simulink model "RemoteMicrogrid"  (R2025a)
settings: Solver=FixedStepAuto  StartTime=0.0  StopTime=8  FixedStep=Ts  MaxStep=1e-3  RelTol=1e-3
PreLoadFcn:
  | RemoteMicrogridInputData
undefined symbols (not defined in the file): BESS, ControlRoom, DiscIntNeverNeededParam, Grid, Load, Machine, Microgrid, MicrogridStatus, PV, relay1, T_on, Ts
libraries: ee_lib x53, fl_lib x39, eeGeneralControl x30, simulink x30, nesl_utility x26, nesl_utility_internal x19, slpidlib x7, eeTransforms x5, eeRmsMeasurement x4, eeTotalHarmonicDistorsion x4, batteryecm_lib x2, simulink_extras x2
(part 3 of 6)

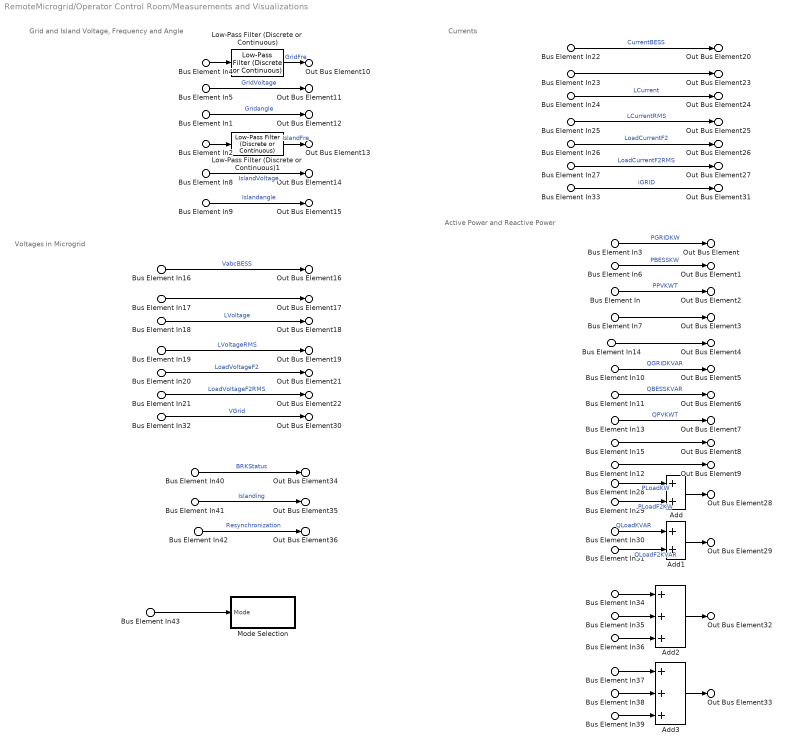
== system RemoteMicrogrid/Operator Control Room/Measurements and Visualizations  ==
  note: Currents
  note: Voltages in Microgrid
  note: Grid and Island Voltage, Frequency and Angle
  note: Active Power and Reactive Power
  Bus Element In4 : Inport  PortName=MGSubstation  Element=MGController.mPLL.Grid.frequency
  Bus Element In5 : Inport  PortName=MGSubstation  Element=MGController.mPLL.Grid.voltage
  Bus Element In1 : Inport  PortName=MGSubstation  Element=MGController.mPLL.Grid.angle
  Bus Element In2 : Inport  PortName=MGSubstation  Element=MGController.mPLL.Island.frequency
  Bus Element In8 : Inport  PortName=MGSubstation  Element=MGController.mPLL.Island.voltage
  Bus Element In9 : Inport  PortName=MGSubstation  Element=MGController.mPLL.Island.angle
  Bus Element In40 : Inport  PortName=MGSubstation  Element=MGController.BRK Status
  Bus Element In41 : Inport  PortName=MGSubstation  Element=MGController.Status.plannedIslanding
  Bus Element In42 : Inport  PortName=MGSubstation  Element=MGController.Status.resync
  Bus Element In43 : Inport  PortName=MGSubstation  Element=MGController.Status.mode
  Bus Element In10 : Inport  PortName=MGSubstation  Element=mPCC.PCC.reactivePower
  Bus Element In37 : Inport  PortName=MGSubstation  Element=mPCC.PCC.reactivePower
  Bus Element In32 : Inport  PortName=MGSubstation  Element=mPCC.PCC.voltage
  Bus Element In33 : Inport  PortName=MGSubstation  Element=mPCC.PCC.current
  Bus Element In3 : Inport  PortName=MGSubstation  Element=mPCC.PCC.activePower
  Bus Element In34 : Inport  PortName=MGSubstation  Element=mPCC.PCC.activePower
  Bus Element In6 : Inport  PortName=MGSubstation  Element=mBESS.active power
  Bus Element In35 : Inport  PortName=MGSubstation  Element=mBESS.active power
  Bus Element In11 : Inport  PortName=MGSubstation  Element=mBESS.reactive power
  Bus Element In38 : Inport  PortName=MGSubstation  Element=mBESS.reactive power
  Bus Element In16 : Inport  PortName=MGSubstation  Element=mBESS.voltage
  Bus Element In22 : Inport  PortName=MGSubstation  Element=mBESS.current
  Bus Element In : Inport  Port=2  PortName=mPV  Element=PV power.PV active power
  Bus Element In36 : Inport  Port=2  PortName=mPV  Element=PV power.PV active power
  Bus Element In13 : Inport  Port=2  PortName=mPV  Element=PV power.PV reactive power
  Bus Element In39 : Inport  Port=2  PortName=mPV  Element=PV power.PV reactive power
  Bus Element In17 : Inport  Port=2  PortName=mPV  Element=PV ac.Va
  Bus Element In23 : Inport  Port=2  PortName=mPV  Element=PV ac.Ia
  Bus Element In7 : Inport  Port=3  PortName=mLoad  Element=active power
  Bus Element In28 : Inport  Port=3  PortName=mLoad  Element=active power
  Bus Element In15 : Inport  Port=3  PortName=mLoad  Element=reactive power
  Bus Element In30 : Inport  Port=3  PortName=mLoad  Element=reactive power
  Bus Element In18 : Inport  Port=3  PortName=mLoad  Element=voltage
  Bus Element In19 : Inport  Port=3  PortName=mLoad  Element=voltageRMS
  Bus Element In24 : Inport  Port=3  PortName=mLoad  Element=current
  Bus Element In25 : Inport  Port=3  PortName=mLoad  Element=currentRMS
  Bus Element In14 : Inport  Port=4  PortName=mLoadF2  Element=active powerF2
  Bus Element In29 : Inport  Port=4  PortName=mLoadF2  Element=active powerF2
  Bus Element In12 : Inport  Port=4  PortName=mLoadF2  Element=reactive powerF2
  Bus Element In31 : Inport  Port=4  PortName=mLoadF2  Element=reactive powerF2
  Bus Element In20 : Inport  Port=4  PortName=mLoadF2  Element=voltageF2
  Bus Element In21 : Inport  Port=4  PortName=mLoadF2  Element=voltageRMSF2
  Bus Element In26 : Inport  Port=4  PortName=mLoadF2  Element=currentF2
  Bus Element In27 : Inport  Port=4  PortName=mLoadF2  Element=currentRMSF2
  Add : Sum
  Add1 : Sum
  Add2 : Sum  Inputs=+++
  Add3 : Sum  Inputs=+++
  Low-Pass Filter (Discrete or Continuous) : eeGeneralControl/Low-Pass Filter (Discrete or Continuous)  K=1  T=0.001  B=inf  A=-inf  init_option=Inherited from block input  x0=0  Ts=-1
  Low-Pass Filter (Discrete or Continuous)1 : eeGeneralControl/Low-Pass Filter (Discrete or Continuous)  K=1  T=0.001  B=inf  A=-inf  init_option=Specify as parameter  x0=0  Ts=-1
  Mode Selection : Subsystem
  Out Bus Element1 : Outport  PortName=Visualization  Element=BESS.activePower
  Out Bus Element6 : Outport  PortName=Visualization  Element=BESS.reactivePower
  Out Bus Element16 : Outport  PortName=Visualization  Element=BESS.voltage
  Out Bus Element20 : Outport  PortName=Visualization  Element=BESS.current
  Out Bus Element2 : Outport  PortName=Visualization  Element=PV.activePower
  Out Bus Element7 : Outport  PortName=Visualization  Element=PV.reactivePower
  Out Bus Element17 : Outport  PortName=Visualization  Element=PV.ACVoltage
  Out Bus Element23 : Outport  PortName=Visualization  Element=PV.ACCurrent
  Out Bus Element3 : Outport  PortName=Visualization  Element=MVLoad.activePower
  Out Bus Element8 : Outport  PortName=Visualization  Element=MVLoad.reactivePower
  Out Bus Element18 : Outport  PortName=Visualization  Element=MVLoad.voltage
  Out Bus Element19 : Outport  PortName=Visualization  Element=MVLoad.voltageRMS
  Out Bus Element24 : Outport  PortName=Visualization  Element=MVLoad.current
  Out Bus Element25 : Outport  PortName=Visualization  Element=MVLoad.currentRMS
  Out Bus Element4 : Outport  PortName=Visualization  Element=LVLoad.activePower
  Out Bus Element9 : Outport  PortName=Visualization  Element=LVLoad.reactivePower
  Out Bus Element21 : Outport  PortName=Visualization  Element=LVLoad.voltage
  Out Bus Element22 : Outport  PortName=Visualization  Element=LVLoad.voltageRMS
  Out Bus Element26 : Outport  PortName=Visualization  Element=LVLoad.current
  Out Bus Element27 : Outport  PortName=Visualization  Element=LVLoad.currentRMS
  Out Bus Element : Outport  PortName=Visualization  Element=Diesel.activePower
  Out Bus Element5 : Outport  PortName=Visualization  Element=Diesel.reactivePower
  Out Bus Element10 : Outport  PortName=Visualization  Element=Diesel.frequency
  Out Bus Element11 : Outport  PortName=Visualization  Element=Diesel.voltage
  Out Bus Element12 : Outport  PortName=Visualization  Element=Diesel.angle
  Out Bus Element13 : Outport  PortName=Visualization  Element=Island.frequency
  Out Bus Element14 : Outport  PortName=Visualization  Element=Island.voltage
  Out Bus Element15 : Outport  PortName=Visualization  Element=Island.angle
  Out Bus Element28 : Outport  PortName=Visualization  Element=Load.activePower
  Out Bus Element29 : Outport  PortName=Visualization  Element=Load.reactivePower
  Out Bus Element30 : Outport  PortName=Visualization  Element=PCC.voltage
  Out Bus Element31 : Outport  PortName=Visualization  Element=PCC.current
  Out Bus Element34 : Outport  PortName=Visualization  Element=PCC.BRKStatus
  Out Bus Element32 : Outport  PortName=Visualization  Element=Generation.activePower
  Out Bus Element33 : Outport  PortName=Visualization  Element=Generation.reactivePower
  Out Bus Element35 : Outport  PortName=Visualization  Element=plannedIslanding
  Out Bus Element36 : Outport  PortName=Visualization  Element=resynchronization
  wires:
  Bus Element In4/1 -> Low-Pass Filter (Discrete or Continuous)/1
  Bus Element In1/1 -> Out Bus Element12/1  "Gridangle"
  Bus Element In9/1 -> Out Bus Element15/1  "Islandangle"
  Bus Element In3/1 -> Out Bus Element/1  "PGRIDKW"
  Bus Element In6/1 -> Out Bus Element1/1  "PBESSKW"
  Bus Element In/1 -> Out Bus Element2/1  "PPVKWT"
  Bus Element In7/1 -> Out Bus Element3/1
  Bus Element In14/1 -> Out Bus Element4/1
  Bus Element In10/1 -> Out Bus Element5/1  "QGRIDKVAR"
  Bus Element In11/1 -> Out Bus Element6/1  "QBESSKVAR"
  Bus Element In13/1 -> Out Bus Element7/1  "QPVKWT"
  Bus Element In15/1 -> Out Bus Element8/1
  Bus Element In12/1 -> Out Bus Element9/1
  Bus Element In5/1 -> Out Bus Element11/1  "GridVoltage"
  Bus Element In2/1 -> Low-Pass Filter (Discrete or Continuous)1/1
  Bus Element In8/1 -> Out Bus Element14/1  "IslandVoltage"
  Bus Element In16/1 -> Out Bus Element16/1  "VabcBESS"
  Bus Element In17/1 -> Out Bus Element17/1
  Bus Element In18/1 -> Out Bus Element18/1  "LVoltage"
  Bus Element In19/1 -> Out Bus Element19/1  "LVoltageRMS"
  Bus Element In20/1 -> Out Bus Element21/1  "LoadVoltageF2"
  Bus Element In21/1 -> Out Bus Element22/1  "LoadVoltageF2RMS"
  Bus Element In23/1 -> Out Bus Element23/1
  Bus Element In24/1 -> Out Bus Element24/1  "LCurrent"
  Bus Element In26/1 -> Out Bus Element26/1  "LoadCurrentF2"
  Bus Element In27/1 -> Out Bus Element27/1  "LoadCurrentF2RMS"
  Bus Element In22/1 -> Out Bus Element20/1  "CurrentBESS"
  Bus Element In25/1 -> Out Bus Element25/1  "LCurrentRMS"
  Bus Element In28/1 -> Add/1  "PLoadKW"
  Bus Element In29/1 -> Add/2  "PLoadF2KW"
  Add/1 -> Out Bus Element28/1
  Add1/1 -> Out Bus Element29/1
  Bus Element In31/1 -> Add1/2  "QLoadF2KVAR"
  Bus Element In30/1 -> Add1/1  "QLoadKVAR"
  Bus Element In32/1 -> Out Bus Element30/1  "VGrid"
  Bus Element In33/1 -> Out Bus Element31/1  "iGRID"
  Bus Element In34/1 -> Add2/1
  Bus Element In35/1 -> Add2/2
  Bus Element In36/1 -> Add2/3
  Bus Element In38/1 -> Add3/2
  Bus Element In39/1 -> Add3/3
  Bus Element In37/1 -> Add3/1
  Add2/1 -> Out Bus Element32/1
  Add3/1 -> Out Bus Element33/1
  Bus Element In40/1 -> Out Bus Element34/1  "BRKStatus"
  Bus Element In41/1 -> Out Bus Element35/1  "Islanding"
  Bus Element In42/1 -> Out Bus Element36/1  "Resynchronization"
  Bus Element In43/1 -> Mode Selection/1(Mode)
  Low-Pass Filter (Discrete or Continuous)/1 -> Out Bus Element10/1  "GridFre"
  Low-Pass Filter (Discrete or Continuous)1/1 -> Out Bus Element13/1  "IslandFre"

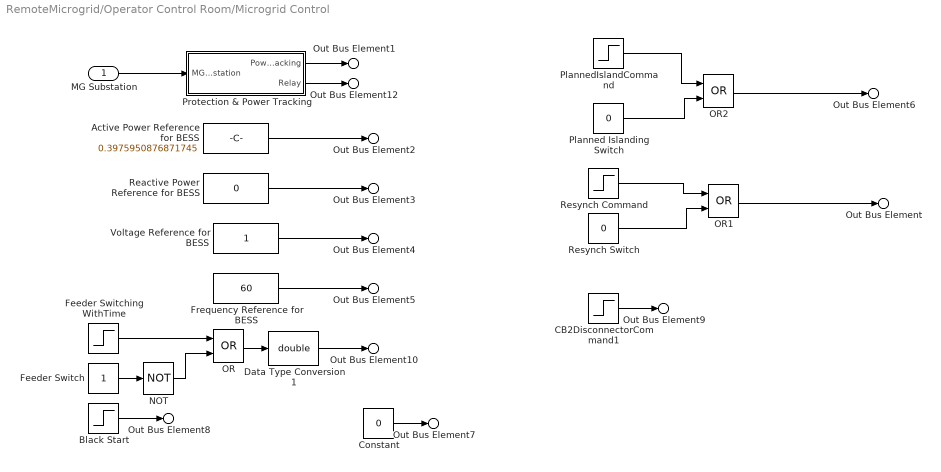
== system RemoteMicrogrid/Operator Control Room/Microgrid Control ==
  MG Substation : Inport
  Active Power Reference for BESS : Constant  Value=0.3975950876871745
  Black Start : Step  Time=100  SampleTime=Ts
  CB2DisconnectorCommand1 : Step  Time=ControlRoom.BRKControl  SampleTime=Ts
  Constant : Constant  Value=0
  Data Type Conversion1 : DataTypeConversion  OutDataTypeStr=double  SaturateOnIntegerOverflow=off  RndMeth=Floor
  Feeder Switch : Constant
  Feeder Switching WithTime : Step  Time=ControlRoom.FeederSwitchTime  SampleTime=Ts
  Frequency Reference for BESS : Constant  Value=60
  NOT : Logic  Operator=NOT  IconShape=distinctive  AllPortsSameDT=off  OutDataTypeStr=boolean
  OR : Logic  Operator=OR  AllPortsSameDT=off  OutDataTypeStr=boolean
  OR1 : Logic  Operator=OR  AllPortsSameDT=off  OutDataTypeStr=boolean
  OR2 : Logic  Operator=OR  AllPortsSameDT=off  OutDataTypeStr=boolean
  Planned Islanding Switch : Constant  Value=0
  PlannedIslandCommand : Step  Time=ControlRoom.PlannedIsland  SampleTime=Ts
  Protection & Power Tracking : Subsystem
  Reactive Power Reference for BESS : Constant  Value=0
  Resynch Command : Step  Time=ControlRoom.Resynch  SampleTime=Ts
  Resynch Switch : Constant  Value=0
  Voltage Reference for BESS : Constant
  Out Bus Element6 : Outport  PortName=CtrlRmSubstation  Element=PlannedIslandCmd
  Out Bus Element9 : Outport  PortName=CtrlRmSubstation  Element=BRKcontrol
  Out Bus Element : Outport  PortName=CtrlRmSubstation  Element=ResynchCmd
  Out Bus Element1 : Outport  PortName=CtrlRmSubstation  Element=PowerCmd
  Out Bus Element2 : Outport  PortName=CtrlRmSubstation  Element=Pref
  Out Bus Element3 : Outport  PortName=CtrlRmSubstation  Element=Qref
  Out Bus Element8 : Outport  PortName=CtrlRmSubstation  Element=BlackStart
  Out Bus Element4 : Outport  PortName=CtrlRmSubstation  Element=Vref
  Out Bus Element5 : Outport  PortName=CtrlRmSubstation  Element=Fref
  Out Bus Element7 : Outport  PortName=CtrlRmSubstation  Element=BESSReactivePower
  Out Bus Element12 : Outport  PortName=CtrlRmSubstation  Element=UnplannedIslanding
  Out Bus Element10 : Outport  Port=2  PortName=CtrlRmFeeder  Element=FeederSwitch
  wires:
  Data Type Conversion1/1 -> Out Bus Element10/1
  Resynch Command/1 -> OR1/1
  OR/1 -> Data Type Conversion1/1
  Active Power Reference for BESS/1 -> Out Bus Element2/1
  PlannedIslandCommand/1 -> OR2/1
  Planned Islanding Switch/1 -> OR2/2
  Resynch Switch/1 -> OR1/2
  Feeder Switching WithTime/1 -> OR/1
  Protection & Power Tracking/1(Power tracking) -> Out Bus Element1/1
  Feeder Switch/1 -> NOT/1
  CB2DisconnectorCommand1/1 -> Out Bus Element9/1
  MG Substation/1 -> Protection & Power Tracking/1(MGSubstation)
  OR2/1 -> Out Bus Element6/1
  Black Start/1 -> Out Bus Element8/1
  Voltage Reference for BESS/1 -> Out Bus Element4/1
  Frequency Reference for BESS/1 -> Out Bus Element5/1
  Constant/1 -> Out Bus Element7/1
  NOT/1 -> OR/2
  OR1/1 -> Out Bus Element/1
  Protection & Power Tracking/2(Relay) -> Out Bus Element12/1
  Reactive Power Reference for BESS/1 -> Out Bus Element3/1

== system RemoteMicrogrid/Operator Control Room/Performance and Power Quality ==
  Bus Element In4 : Inport  PortName=Visualization  Element=MVLoad.voltage
  Bus Element In5 : Inport  PortName=Visualization  Element=MVLoad.current
  Bus Element In7 : Inport  PortName=Visualization  Element=MVLoad.voltageRMS
  Bus Element In8 : Inport  PortName=Visualization  Element=MVLoad.currentRMS
  Bus Element In9 : Inport  PortName=Visualization  Element=MVLoad.activePower
  Bus Element In1 : Inport  PortName=Visualization  Element=PCC.voltage
  Bus Element In6 : Inport  PortName=Visualization  Element=PCC.current
  Bus Element In2 : Inport  PortName=Visualization  Element=Island.frequency
  Bus Element In3 : Inport  PortName=Visualization  Element=Island.voltage
  Bus Element In10 : Inport  PortName=Visualization  Element=Generation.activePower
  Bus Element In11 : Inport  PortName=Visualization  Element=Generation.reactivePower
  Bus Element In12 : Inport  PortName=Visualization  Element=Load.activePower
  Bus Element In13 : Inport  PortName=Visualization  Element=Load.reactivePower
  "Load Performance " : Subsystem
  Loss Calculation : Subsystem
  "Microgrid Power Quality " : Subsystem
  THD : Subsystem
  wires:
  Bus Element In4/1 -> THD/1(LoadVoltage)
  Bus Element In5/1 -> THD/2(LoadCurrent)
  Bus Element In1/1 -> THD/3(PCCVoltage)
  Bus Element In6/1 -> THD/4(PCCCurrent)
  Bus Element In2/1 -> "Microgrid Power Quality "/1(Frequency)
  Bus Element In3/1 -> "Microgrid Power Quality "/2(Voltage)
  Bus Element In7/1 -> "Load Performance "/1(VRMS)
  Bus Element In8/1 -> "Load Performance "/2(IRMS)
  Bus Element In9/1 -> "Load Performance "/3(Active Power)
  Bus Element In10/1 -> Loss Calculation/1(Active Power Gen)
  Bus Element In11/1 -> Loss Calculation/2(Reactive Power Gen)
  Bus Element In12/1 -> Loss Calculation/3(Active Power Load)
  Bus Element In13/1 -> Loss Calculation/4(Reactive Power Load)

== system RemoteMicrogrid/PV /30 kW PV ==
  In Bus Element : Inport  PortName=PV
  Current and Voltage Sensor (Three-Phase)2 : ee_lib/Sensors & Transducers/Current and Voltage Sensor (Three-Phase)  vMeasurementType=ee.enum.vmeasurement.lg  outputUnit=ee.enum.unit.pu  SRated=PV.MVA_base_new A*V  VRated=PV.KV_base_new V  I_specify=off  I_priority=None  I=[0, 0, 0] A  I_nominal_specify=off  I_nominal_value=1  I_nominal_unit=A  V_specify=off  V_priority=None  V=[0, 0, 0] V  V_nominal_specify=off  V_nominal_value=1  V_nominal_unit=V
      settings: InternalSimscapePortConfiguration="{\"Bottom\":[],\"Left\":[{\"id\":\"N1\",\"label\":\"~1\",\"type\":\"foundation.electrical.three_phase\"}],\"Right\":[{\"id\":\"V_output\",\"label\":\"V\",\"type\":\"output\"},{\"id\":\"I_output\",\"label\":\"I\",\"type\":\"output\"},{\"id\":\"N2\",\"label\":\"~2\",\"type\":\"foundation.electrical.three_phase\"}],\"Top\":[]}"
  L Filter1 : Subsystem
  Measurement1 : Subsystem
  PS-Simulink Converter1 : nesl_utility/PS-Simulink Converter  PhysicalDomain=network_engine_domain  SubClassName=ps_output  LeftPortType=input  RightPortType=output  PseudoPeriodic=off  Frequencies=[]  VectorFormat=inherit  Unit=inherit  AffineConversion=off
  PS-Simulink Converter3 : nesl_utility/PS-Simulink Converter  PhysicalDomain=network_engine_domain  SubClassName=ps_output  LeftPortType=input  RightPortType=output  PseudoPeriodic=off  Frequencies=[]  VectorFormat=inherit  Unit=inherit  AffineConversion=off
  PV Inverter 2 : Subsystem
  Terminator : Terminator
  ~ : PMIOPort  Side=Left
  PV power : Outport
  wires:
  PS-Simulink Converter3/1 -> Terminator/1
  In Bus Element/1 -> PV Inverter 2/1(PV)
  Measurement1/1(ipv1) -> PV Inverter 2/2(ipv1)
  PV Inverter 2/1(PV power) -> PV power/1
  PS-Simulink Converter1/1 -> Measurement1/1(u)
  connections:
  PV Inverter 2/RConn1 -- L Filter1/LConn1
  PS-Simulink Converter3/LConn1 -- Current and Voltage Sensor (Three-Phase)2/RConn1
  PS-Simulink Converter1/LConn1 -- Current and Voltage Sensor (Three-Phase)2/RConn2
  ~/RConn1 -- Current and Voltage Sensor (Three-Phase)2/RConn3
  Current and Voltage Sensor (Three-Phase)2/LConn1 -- L Filter1/RConn1

== system RemoteMicrogrid/PV /PLL & Measurements ==
  V : Inport
  Measurement2 : Subsystem
  Subsystem : Subsystem
  Out Bus Element : Outport  PortName=PV  Element=Vq
  Out Bus Element1 : Outport  PortName=PV  Element=Vd
  Out Bus Element2 : Outport  PortName=PV  Element=w
  Out Bus Element3 : Outport  PortName=PV  Element=Theta
  Out Bus Element4 : Outport  PortName=PV  Element=Vmag
  wires:
  V/1 -> Measurement2/1(u)
  Subsystem/2(freq) -> Out Bus Element2/1
  Subsystem/5(Vq) -> Out Bus Element/1
  Subsystem/3(angle) -> Out Bus Element3/1
  Subsystem/4(Vd) -> Out Bus Element1/1
  Measurement2/1(Vg) -> Subsystem/1(abc)
  Subsystem/1(mag) -> Out Bus Element4/1

== system RemoteMicrogrid/Diesel Substation, BESS, & Microgrid Controller/BESS and Controller/BESS ==
  Average-Value Voltage Source Converter (Three-Phase) : ee_lib/Semiconductors & Converters/Converters/Average-Value Voltage Source Converter (Three-Phase)  port_option=ee.enum.threePhasePort.expanded  frequency_option=ee.enum.converters.frequency.variable  input_option=ee.enum.converters.inputOption.ModWave  FRated=60 Hz  losses_parameterization=ee.enum.converters.losses.fixed  Pfixed=1 W  ks=0.01  kc1=1.7 V  kc2=0.01 Ohm  Ploss_vect=[100, 800, 1870, 3250, 4900] W  Irms_vect=[10, 100, 200, 300, 400] A  Vdc_nom=300 V  thermal_mass=30000 J/K  temperature_specify=off  temperature_priority=High  temperature=298.15 K  temperature_nominal_specify=off  temperature_nominal_value=1  temperature_nominal_unit=K
      settings: InternalSimscapePortConfiguration="{\"Bottom\":[],\"Left\":[{\"id\":\"ModWave\",\"label\":\"ModWave\",\"type\":\"input\"},{\"id\":\"a\",\"label\":\"a\",\"type\":\"foundation.electrical.electrical\"},{\"id\":\"b\",\"label\":\"b\",\"type\":\"foundation.electrical.electrical\"},{\"id\":\"c\",\"label\":\"c\",\"type\":\"foundation.electrical.electrical\"}],\"Right\":[{\"id\":\"p\",\"label\":\"+\",\"type\":\"foundation.electrical.electrical\"},{\"id\":\"n\",\"label\":\"-\",\"type\":\"foundation.electrical.electrical\"}],\"Top\":[]}"
  Battery : batteryecm_lib/Battery  Vnom=BESS.Vdc V  prm_dir=simscape.enum.battery.prm_dir.disabled  R1_dis=2 Ohm  R1_ch=2 Ohm  R1=BESS.Rs Ohm  prm_AH=simscape.enum.battery.prm_AH.infinite  AH=50 A*hr  V1=11.5 V  AH1=25 A*hr  prm_R2=simscape.enum.battery.prm_R2.disabled  R2=2000 Ohm  Tmeas=298.15 K  charge_measurement_port=simscape.enum.battery.enable.no  prm_dyn=simscape.enum.battery.prm_dyn.off  Rp1=0.005 Ohm  tau1=30 s  Rp2=0.005 Ohm  tau2=30 s  Rp3=0.005 Ohm  tau3=30 s  Rp4=0.005 Ohm  tau4=30 s  Rp5=0.005 Ohm  tau5=30 s  prm_fade=simscape.enum.battery.prm_fade.disabled  N_fade=100  AH_fade=45 A*hr  R1_fade=2.02 Ohm  R1_ch_fade=2.02 Ohm  V1_fade=10.35 V  prm_age=simscape.enum.battery.prm_age.disabled  prm_age_OCV=simscape.enum.battery.prm_age_OCV.OCV  OCV_age=0.9  SOC_age=60  Tmeas_age=298.15 K  delta_time_age_vec=[0] d  temperature_age_vec=[273] K  OCV_scaling_age=2.2134e6  OCV_offset_age=1.632e6  temp_exp_age=0.515833569 V  t_exp_age=0.75  Vnom_T2=12 V  R1_T2=2.2 Ohm  R1_T2_dis=2.2 Ohm  R1_T2_ch=2.2 Ohm  V1_T2=11.4 V  R2_T2=2200 Ohm  Rp1_T2=0.005 Ohm  tau1_T2=30 s  Rp2_T2=0.005 Ohm  tau2_T2=30 s  Rp3_T2=0.005 Ohm  tau3_T2=30 s  Rp4_T2=0.005 Ohm  tau4_T2=30 s  Rp5_T2=0.005 Ohm  tau5_T2=30 s  Tmeas2=273.15 K  thermal_port=simscape.enum.thermaleffects.omit  thermal_mass=30000 J/K  i_specify=off  i_priority=None  i=0 A  i_nominal_specify=off  i_nominal_value=1  i_nominal_unit=A  v_specify=off  v_priority=None  v=0 V  v_nominal_specify=off  v_nominal_value=1  v_nominal_unit=V  charge_specify=off  charge_priority=High  charge=50 A*hr  charge_nominal_specify=off  charge_nominal_value=1  charge_nominal_unit=A*hr  num_cycles_specify=off  num_cycles_priority=High  num_cycles=0  num_cycles_nominal_specify=off  num_cycles_nominal_value=1  num_cycles_nominal_unit=1  temperature_specify=off  temperature_priority=High  temperature=298.15 K  temperature_nominal_specify=off  temperature_nominal_value=1  temperature_nominal_unit=K
  Battery1 : batteryecm_lib/Battery  Vnom=BESS.Vdc V  prm_dir=simscape.enum.battery.prm_dir.disabled  R1_dis=2 Ohm  R1_ch=2 Ohm  R1=BESS.Rs Ohm  prm_AH=simscape.enum.battery.prm_AH.infinite  AH=50 A*hr  V1=11.5 V  AH1=25 A*hr  prm_R2=simscape.enum.battery.prm_R2.disabled  R2=2000 Ohm  Tmeas=298.15 K  charge_measurement_port=simscape.enum.battery.enable.no  prm_dyn=simscape.enum.battery.prm_dyn.off  Rp1=0.005 Ohm  tau1=30 s  Rp2=0.005 Ohm  tau2=30 s  Rp3=0.005 Ohm  tau3=30 s  Rp4=0.005 Ohm  tau4=30 s  Rp5=0.005 Ohm  tau5=30 s  prm_fade=simscape.enum.battery.prm_fade.disabled  N_fade=100  AH_fade=45 A*hr  R1_fade=2.02 Ohm  R1_ch_fade=2.02 Ohm  V1_fade=10.35 V  prm_age=simscape.enum.battery.prm_age.disabled  prm_age_OCV=simscape.enum.battery.prm_age_OCV.OCV  OCV_age=0.9  SOC_age=60  Tmeas_age=298.15 K  delta_time_age_vec=[0] d  temperature_age_vec=[273] K  OCV_scaling_age=2.2134e6  OCV_offset_age=1.632e6  temp_exp_age=0.515833569 V  t_exp_age=0.75  Vnom_T2=12 V  R1_T2=2.2 Ohm  R1_T2_dis=2.2 Ohm  R1_T2_ch=2.2 Ohm  V1_T2=11.4 V  R2_T2=2200 Ohm  Rp1_T2=0.005 Ohm  tau1_T2=30 s  Rp2_T2=0.005 Ohm  tau2_T2=30 s  Rp3_T2=0.005 Ohm  tau3_T2=30 s  Rp4_T2=0.005 Ohm  tau4_T2=30 s  Rp5_T2=0.005 Ohm  tau5_T2=30 s  Tmeas2=273.15 K  thermal_port=simscape.enum.thermaleffects.omit  thermal_mass=30000 J/K  i_specify=off  i_priority=None  i=0 A  i_nominal_specify=off  i_nominal_value=1  i_nominal_unit=A  v_specify=off  v_priority=None  v=0 V  v_nominal_specify=off  v_nominal_value=1  v_nominal_unit=V  charge_specify=off  charge_priority=High  charge=50 A*hr  charge_nominal_specify=off  charge_nominal_value=1  charge_nominal_unit=A*hr  num_cycles_specify=off  num_cycles_priority=High  num_cycles=0  num_cycles_nominal_specify=off  num_cycles_nominal_value=1  num_cycles_nominal_unit=1  temperature_specify=off  temperature_priority=High  temperature=298.15 K  temperature_nominal_specify=off  temperature_nominal_value=1  temperature_nominal_unit=K
  DC Voltage Source : fl_lib/Electrical/Electrical Sources/DC Voltage Source  Commented=on  v0=BESS.Vdc*2 V
  Electrical Reference : fl_lib/Electrical/Electrical Elements/Electrical Reference  Commented=on
  Electrical Reference4 : fl_lib/Electrical/Electrical Elements/Electrical Reference
  Phase Splitter : ee_lib/Connectors & References/Phase Splitter
  Voltage Sensor : fl_lib/Electrical/Electrical Sensors/Voltage Sensor  Commented=on
  Modulation : PMIOPort  Side=Left
  ~ : PMIOPort  Port=2  Side=Left
  connections:
  Battery/LConn1 -- Voltage Sensor/LConn1 -- DC Voltage Source/LConn1 -- Average-Value Voltage Source Converter (Three-Phase)/RConn1
  Battery/RConn1 -- Electrical Reference4/LConn1 -- Battery1/LConn1
  Phase Splitter/RConn3 -- Average-Value Voltage Source Converter (Three-Phase)/LConn4
  Battery1/RConn1 -- Voltage Sensor/RConn2 -- Electrical Reference/LConn1 -- DC Voltage Source/RConn1 -- Average-Value Voltage Source Converter (Three-Phase)/RConn2
  Phase Splitter/RConn1 -- Average-Value Voltage Source Converter (Three-Phase)/LConn2
  Modulation/RConn1 -- Average-Value Voltage Source Converter (Three-Phase)/LConn1
  Phase Splitter/RConn2 -- Average-Value Voltage Source Converter (Three-Phase)/LConn3
  Phase Splitter/LConn1 -- ~/RConn1

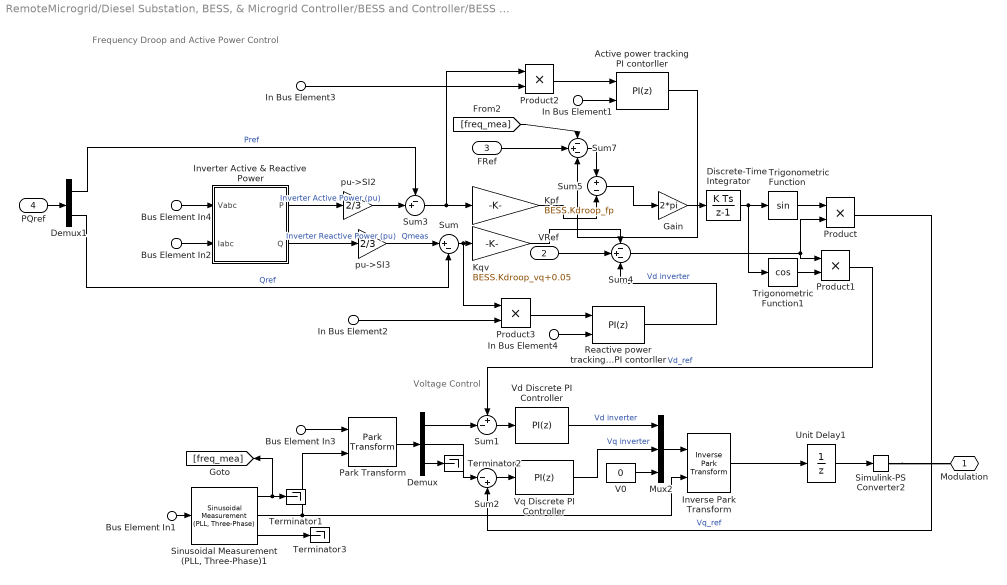
== system RemoteMicrogrid/Diesel Substation, BESS, & Microgrid Controller/BESS and Controller/BESS Control ==
  note: Frequency Droop and Active Power Control
  note: Voltage Control
  Bus Element In1 : Inport  PortName=mBESS  Element=voltage
  Bus Element In3 : Inport  PortName=mBESS  Element=voltage
  Bus Element In4 : Inport  PortName=mBESS  Element=voltage
  Bus Element In2 : Inport  PortName=mBESS  Element=current
  VRef : Inport  Port=2
  FRef : Inport  Port=3
  PQref : Inport  Port=4
  In Bus Element2 : Inport  Port=5  PortName=CntrlRmSubstation  Element=PowerCmd
  In Bus Element3 : Inport  Port=5  PortName=CntrlRmSubstation  Element=PowerCmd
  In Bus Element1 : Inport  Port=5  PortName=CntrlRmSubstation  Element=UnplannedIslanding
  In Bus Element4 : Inport  Port=5  PortName=CntrlRmSubstation  Element=UnplannedIslanding
  Active power tracking PI contorller : slpidlib/PID Controller  Controller=PI  Form=Parallel  TimeDomain=Discrete-time  UseExternalTs=off  SampleTime=Ts  IntegratorMethod=Forward Euler  FilterMethod=Forward Euler  ControllerParametersSource=internal  P=Kp_P  I=Ki_P  UseKiTs=off  D=0  UseExternalDerivativeSource=off  N=100  UseFilter=on  TunerSelectOption=Transfer Function Based (PID Tuner App)  ZeroCross=off  InitialConditionSource=internal  InitialConditionForIntegrator=BESS.Kp_0*0  InitialConditionForFilter=0  DifferentiatorICPrevScaledInput=0  ExternalReset=rising  TrackingMode=off  Kt=1  LimitOutput=off  SatLimitsSource=internal  UpperSaturationLimit=0.2  LowerSaturationLimit=-0.2  LinearizeAsGain=on  AntiWindupMode=none  Kb=1  LimitIntegrator=off  UpperIntegratorSaturationLimit=inf  LowerIntegratorSaturationLimit=-inf  POutMin=[]  POutMax=[]  IOutMin=[]  IOutMax=[]  DOutMin=[]  DOutMax=[]  NOutMin=[]  NOutMax=[]  SumOutMin=[]  SumOutMax=[]  SaturationOutMin=[]  SaturationOutMax=[]  PParamMin=[]  PParamMax=[]  IParamMin=[]  IParamMax=[]  DParamMin=[]  DParamMax=[]  NParamMin=[]  NParamMax=[]  KbParamMin=[]  KbParamMax=[]  KtParamMin=[]  KtParamMax=[]  KbOutMin=[]  KbOutMax=[]  KtOutMin=[]  KtOutMax=[]  IntegratorOutMin=[]  IntegratorOutMax=[]  FilterOutMin=[]  FilterOutMax=[]  SumI1OutMin=[]  SumI1OutMax=[]  SumI2OutMin=[]  SumI2OutMax=[]  SumI3OutMin=[]  SumI3OutMax=[]  SumI4OutMin=[]  SumI4OutMax=[]  SumDOutMin=[]  SumDOutMax=[]  DifferentiatorOutMin=[]  DifferentiatorOutMax=[]  FilterDiffOutCoefMin=[]  FilterDiffOutCoefMax=[]  ReciprocalOutMin=[]  ReciprocalOutMax=[]  SumDenOutMin=[]  SumDenOutMax=[]  SumNumOutMin=[]  SumNumOutMax=[]  DivideOutMin=[]  DivideOutMax=[]  UdiffTsProdOutMin=[]  UdiffTsProdOutMax=[]  NTsProdOutMin=[]  NTsProdOutMax=[]  UintegralTsProdOutMin=[]  UintegralTsProdOutMax=[]  UngainTsProdOutMin=[]  UngainTsProdOutMax=[]  ClampingZeroOutDataTypeStr=Inherit: Inherit via back propagation  ClampingZeroOutMin=[]  ClampingZeroOutMax=[]  FilterDenConstantOutDataTypeStr=Inherit: Inherit via back propagation  FilterDenConstantOutMin=[]  FilterDenConstantOutMax=[]  PCopyOutDataTypeStr=Inherit: Inherit via back propagation  PCopyOutMin=[]  PCopyOutMax=[]  NCopyOutDataTypeStr=Inherit: Inherit via back propagation  NCopyOutMin=[]  NCopyOutMax=[]  IntegratorContinuousStateAttributes=''  IntegratorStateMustResolveToSignalObject=off  IntegratorRTWStateStorageClass=Auto  FilterContinuousStateAttributes=''  FilterStateMustResolveToSignalObject=off  FilterRTWStateStorageClass=Auto  ParallelPVariant=InternalParameters  IdealPVariant=Disabled  IVariant=InternalParameters  DVariant=Disabled  IntegratorVariant=Discrete  SatVariant=Disabled  AWVariant=Passthrough  PCopyVariant=Disabled  TRVariant=Disabled  FdbkBlocksVariant=Forward  IdealPFdbkVariant=Disabled  SatFdbkVariant=Disabled  DerivativeFilterVariant=Disabled  NVariant=Disabled  NCopyVariant=Disabled_SignalSpec  FilterICVariant=Disabled  IntegratorICVariant=InternalICs  ExternalResetVariant=ExternalReset  TRSumVariant=Passthrough  SumFdbkVariant=Disabled  SumVariant=Sum_PI  TsampFilterVariant=InternalTs  TsampNgainVariant=Passthrough  TsampIntegralVariant=Disabled_SignalSpec  ExternalSaturationOutDataTypeStr=Inherit: Same as second input  DerivativeSourceVariant=Disabled  PreIntVariant=InternalPreInt
  Demux : Demux  Outputs=3
  Demux1 : Demux  Outputs=2
  Discrete-Time Integrator : DiscreteIntegrator  SampleTime=Ts  ICPrevOutput=DiscIntNeverNeededParam  ICPrevScaledInput=DiscIntNeverNeededParam
  Gain : Gain  Gain=2*pi
  Inverse Park Transform : eeTransforms/Inverse Park Transform  AxisAlignment=Q-axis  PowerInvariant=off
  "Inverter Active & Reactive Power " : Subsystem
  Kpf : Gain  Gain=BESS.Kdroop_fp
  Kqv : Gain  Gain=BESS.Kdroop_vq+0.05
  Mux2 : Mux  Inputs=3
  Park Transform : eeTransforms/Park Transform  AxisAlignment=Q-axis  PowerInvariant=off
  Product{,1..3} (4 alike) : Product
  Reactive power tracking PI contorller : slpidlib/PID Controller  Controller=PI  Form=Parallel  TimeDomain=Discrete-time  UseExternalTs=off  SampleTime=Ts  IntegratorMethod=Forward Euler  FilterMethod=Forward Euler  ControllerParametersSource=internal  P=Kp_Q  I=Ki_Q  UseKiTs=off  D=0  UseExternalDerivativeSource=off  N=100  UseFilter=on  TunerSelectOption=Transfer Function Based (PID Tuner App)  InitialConditionSource=internal  InitialConditionForIntegrator=BESS.Kq_0  InitialConditionForFilter=0  DifferentiatorICPrevScaledInput=0  ExternalReset=rising  TrackingMode=off  Kt=1  LimitOutput=off  SatLimitsSource=internal  UpperSaturationLimit=1.2  LowerSaturationLimit=0  LinearizeAsGain=on  AntiWindupMode=none  Kb=1  LimitIntegrator=off  UpperIntegratorSaturationLimit=inf  LowerIntegratorSaturationLimit=-inf  POutMin=[]  POutMax=[]  IOutMin=[]  IOutMax=[]  DOutMin=[]  DOutMax=[]  NOutMin=[]  NOutMax=[]  SumOutMin=[]  SumOutMax=[]  SaturationOutMin=[]  SaturationOutMax=[]  PParamMin=[]  PParamMax=[]  IParamMin=[]  IParamMax=[]  DParamMin=[]  DParamMax=[]  NParamMin=[]  NParamMax=[]  KbParamMin=[]  KbParamMax=[]  KtParamMin=[]  KtParamMax=[]  KbOutMin=[]  KbOutMax=[]  KtOutMin=[]  KtOutMax=[]  IntegratorOutMin=[]  IntegratorOutMax=[]  FilterOutMin=[]  FilterOutMax=[]  SumI1OutMin=[]  SumI1OutMax=[]  SumI2OutMin=[]  SumI2OutMax=[]  SumI3OutMin=[]  SumI3OutMax=[]  SumI4OutMin=[]  SumI4OutMax=[]  SumDOutMin=[]  SumDOutMax=[]  DifferentiatorOutMin=[]  DifferentiatorOutMax=[]  FilterDiffOutCoefMin=[]  FilterDiffOutCoefMax=[]  ReciprocalOutMin=[]  ReciprocalOutMax=[]  SumDenOutMin=[]  SumDenOutMax=[]  SumNumOutMin=[]  SumNumOutMax=[]  DivideOutMin=[]  DivideOutMax=[]  UdiffTsProdOutMin=[]  UdiffTsProdOutMax=[]  NTsProdOutMin=[]  NTsProdOutMax=[]  UintegralTsProdOutMin=[]  UintegralTsProdOutMax=[]  UngainTsProdOutMin=[]  UngainTsProdOutMax=[]  ClampingZeroOutDataTypeStr=Inherit: Inherit via back propagation  ClampingZeroOutMin=[]  ClampingZeroOutMax=[]  FilterDenConstantOutDataTypeStr=Inherit: Inherit via back propagation  FilterDenConstantOutMin=[]  FilterDenConstantOutMax=[]  PCopyOutDataTypeStr=Inherit: Inherit via back propagation  PCopyOutMin=[]  PCopyOutMax=[]  NCopyOutDataTypeStr=Inherit: Inherit via back propagation  NCopyOutMin=[]  NCopyOutMax=[]  IntegratorContinuousStateAttributes=''  IntegratorStateMustResolveToSignalObject=off  IntegratorRTWStateStorageClass=Auto  FilterContinuousStateAttributes=''  FilterStateMustResolveToSignalObject=off  FilterRTWStateStorageClass=Auto  ParallelPVariant=InternalParameters  IdealPVariant=Disabled  IVariant=InternalParameters  DVariant=Disabled  IntegratorVariant=Discrete  SatVariant=Disabled  AWVariant=Passthrough  PCopyVariant=Disabled  TRVariant=Disabled  FdbkBlocksVariant=Forward  IdealPFdbkVariant=Disabled  SatFdbkVariant=Disabled  DerivativeFilterVariant=Disabled  NVariant=Disabled  NCopyVariant=Disabled_SignalSpec  FilterICVariant=Disabled  IntegratorICVariant=InternalICs  ExternalResetVariant=ExternalReset  TRSumVariant=Passthrough  SumFdbkVariant=Disabled  SumVariant=Sum_PI  TsampFilterVariant=InternalTs  TsampNgainVariant=Passthrough  TsampIntegralVariant=Disabled_SignalSpec  ExternalSaturationOutDataTypeStr=Inherit: Same as second input  DerivativeSourceVariant=Disabled  PreIntVariant=InternalPreInt
  Simulink-PS Converter2 : nesl_utility_internal/Simulink-PS Converter  PhysicalDomain=network_engine_domain  SubClassName=ps_input  LeftPortType=input  RightPortType=output  PseudoPeriodic=off  Frequencies=[]  NoiseDistribution=none  NoiseParameters=[]  Unit=1  AffineConversion=off  FilteringAndDerivatives=provide  SimscapeFilterOrder=1  InputFilterTimeConstant=0.001  UdotUserProvided=0
  "Sinusoidal Measurement (PLL, Three-Phase)1" : eeSinusoidalMeasurement/Sinusoidal Measurement (PLL, Three-Phase)  Kp_LF=BESS.PLL_Kp  Ki_LF=BESS.PLL_Ki  F0=Grid.Frequency  Theta0=0  Ts=Ts
  Sum : Sum  Inputs=|+-
  Sum1 : Sum  Inputs=+-|  InputSameDT=on  SaturateOnIntegerOverflow=on  OutDataTypeStr=Inherit: Same as first input
  Sum2 : Sum  Inputs=|-+  InputSameDT=on  SaturateOnIntegerOverflow=on  OutDataTypeStr=Inherit: Same as first input
  Sum3 : Sum  Inputs=-+|
  Sum4 : Sum  Inputs=-+-
  Sum5 : Sum  Inputs=+-
  Sum7 : Sum  Inputs=-+-
  Terminator1 : Terminator
  Terminator2 : Terminator
  Terminator3 : Terminator
  Trigonometric Function : Trigonometry
  Trigonometric Function1 : Trigonometry  Operator=cos
  Unit Delay1 : UnitDelay  SampleTime=Ts  HasFrameUpgradeWarning=on
  V0 : Constant  Value=0
  Vd Discrete PI Controller : slpidlib/PID Controller  Controller=PI  Form=Parallel  TimeDomain=Discrete-time  UseExternalTs=off  SampleTime=Ts  IntegratorMethod=Forward Euler  FilterMethod=Forward Euler  ControllerParametersSource=internal  P=Kp_vd  I=Ki_vd  UseKiTs=off  D=0  UseExternalDerivativeSource=off  N=100  UseFilter=on  TunerSelectOption=Transfer Function Based (PID Tuner App)  InitialConditionSource=internal  InitialConditionForIntegrator=0.35  InitialConditionForFilter=0  DifferentiatorICPrevScaledInput=0  ExternalReset=none  TrackingMode=off  Kt=1  LimitOutput=on  SatLimitsSource=internal  UpperSaturationLimit=1.1  LowerSaturationLimit=-1.1  LinearizeAsGain=on  AntiWindupMode=none  Kb=1  LimitIntegrator=off  UpperIntegratorSaturationLimit=inf  LowerIntegratorSaturationLimit=-inf  POutMin=[]  POutMax=[]  IOutMin=[]  IOutMax=[]  DOutMin=[]  DOutMax=[]  NOutMin=[]  NOutMax=[]  SumOutMin=[]  SumOutMax=[]  SaturationOutMin=[]  SaturationOutMax=[]  PParamMin=[]  PParamMax=[]  IParamMin=[]  IParamMax=[]  DParamMin=[]  DParamMax=[]  NParamMin=[]  NParamMax=[]  KbParamMin=[]  KbParamMax=[]  KtParamMin=[]  KtParamMax=[]  KbOutMin=[]  KbOutMax=[]  KtOutMin=[]  KtOutMax=[]  IntegratorOutMin=[]  IntegratorOutMax=[]  FilterOutMin=[]  FilterOutMax=[]  SumI1OutMin=[]  SumI1OutMax=[]  SumI2OutMin=[]  SumI2OutMax=[]  SumI3OutMin=[]  SumI3OutMax=[]  SumI4OutMin=[]  SumI4OutMax=[]  SumDOutMin=[]  SumDOutMax=[]  DifferentiatorOutMin=[]  DifferentiatorOutMax=[]  FilterDiffOutCoefMin=[]  FilterDiffOutCoefMax=[]  ReciprocalOutMin=[]  ReciprocalOutMax=[]  SumDenOutMin=[]  SumDenOutMax=[]  SumNumOutMin=[]  SumNumOutMax=[]  DivideOutMin=[]  DivideOutMax=[]  UdiffTsProdOutMin=[]  UdiffTsProdOutMax=[]  NTsProdOutMin=[]  NTsProdOutMax=[]  UintegralTsProdOutMin=[]  UintegralTsProdOutMax=[]  UngainTsProdOutMin=[]  UngainTsProdOutMax=[]  ClampingZeroOutDataTypeStr=Inherit: Inherit via back propagation  ClampingZeroOutMin=[]  ClampingZeroOutMax=[]  FilterDenConstantOutDataTypeStr=Inherit: Inherit via back propagation  FilterDenConstantOutMin=[]  FilterDenConstantOutMax=[]  PCopyOutDataTypeStr=Inherit: Inherit via back propagation  PCopyOutMin=[]  PCopyOutMax=[]  NCopyOutDataTypeStr=Inherit: Inherit via back propagation  NCopyOutMin=[]  NCopyOutMax=[]  IntegratorContinuousStateAttributes=''  IntegratorStateMustResolveToSignalObject=off  IntegratorRTWStateStorageClass=Auto  FilterContinuousStateAttributes=''  FilterStateMustResolveToSignalObject=off  FilterRTWStateStorageClass=Auto  ParallelPVariant=InternalParameters  IdealPVariant=Disabled  IVariant=InternalParameters  DVariant=Disabled  IntegratorVariant=Discrete  SatVariant=Enabled  AWVariant=Passthrough  PCopyVariant=Disabled  TRVariant=Disabled  FdbkBlocksVariant=Forward  IdealPFdbkVariant=Disabled  SatFdbkVariant=Disabled  DerivativeFilterVariant=Disabled  NVariant=Disabled  NCopyVariant=Disabled_SignalSpec  FilterICVariant=Disabled  IntegratorICVariant=InternalICs  ExternalResetVariant=Disabled  TRSumVariant=Passthrough  SumFdbkVariant=Disabled  SumVariant=Sum_PI  TsampFilterVariant=InternalTs  TsampNgainVariant=Passthrough  TsampIntegralVariant=Disabled_SignalSpec  ExternalSaturationOutDataTypeStr=Inherit: Same as second input  DerivativeSourceVariant=Disabled  PreIntVariant=InternalPreInt
  Vq Discrete PI Controller : slpidlib/PID Controller  Controller=PI  Form=Parallel  TimeDomain=Discrete-time  UseExternalTs=off  SampleTime=Ts  IntegratorMethod=Forward Euler  FilterMethod=Forward Euler  ControllerParametersSource=internal  P=Kp_vq  I=Ki_vq  UseKiTs=off  D=0  UseExternalDerivativeSource=off  N=100  UseFilter=on  TunerSelectOption=Transfer Function Based (PID Tuner App)  InitialConditionSource=internal  InitialConditionForIntegrator=0.44  InitialConditionForFilter=0  DifferentiatorICPrevScaledInput=0  ExternalReset=none  TrackingMode=off  Kt=1  LimitOutput=on  SatLimitsSource=internal  UpperSaturationLimit=1.1  LowerSaturationLimit=-1.1  LinearizeAsGain=on  AntiWindupMode=none  Kb=1  LimitIntegrator=off  UpperIntegratorSaturationLimit=inf  LowerIntegratorSaturationLimit=-inf  POutMin=[]  POutMax=[]  IOutMin=[]  IOutMax=[]  DOutMin=[]  DOutMax=[]  NOutMin=[]  NOutMax=[]  SumOutMin=[]  SumOutMax=[]  SaturationOutMin=[]  SaturationOutMax=[]  PParamMin=[]  PParamMax=[]  IParamMin=[]  IParamMax=[]  DParamMin=[]  DParamMax=[]  NParamMin=[]  NParamMax=[]  KbParamMin=[]  KbParamMax=[]  KtParamMin=[]  KtParamMax=[]  KbOutMin=[]  KbOutMax=[]  KtOutMin=[]  KtOutMax=[]  IntegratorOutMin=[]  IntegratorOutMax=[]  FilterOutMin=[]  FilterOutMax=[]  SumI1OutMin=[]  SumI1OutMax=[]  SumI2OutMin=[]  SumI2OutMax=[]  SumI3OutMin=[]  SumI3OutMax=[]  SumI4OutMin=[]  SumI4OutMax=[]  SumDOutMin=[]  SumDOutMax=[]  DifferentiatorOutMin=[]  DifferentiatorOutMax=[]  FilterDiffOutCoefMin=[]  FilterDiffOutCoefMax=[]  ReciprocalOutMin=[]  ReciprocalOutMax=[]  SumDenOutMin=[]  SumDenOutMax=[]  SumNumOutMin=[]  SumNumOutMax=[]  DivideOutMin=[]  DivideOutMax=[]  UdiffTsProdOutMin=[]  UdiffTsProdOutMax=[]  NTsProdOutMin=[]  NTsProdOutMax=[]  UintegralTsProdOutMin=[]  UintegralTsProdOutMax=[]  UngainTsProdOutMin=[]  UngainTsProdOutMax=[]  ClampingZeroOutDataTypeStr=Inherit: Inherit via back propagation  ClampingZeroOutMin=[]  ClampingZeroOutMax=[]  FilterDenConstantOutDataTypeStr=Inherit: Inherit via back propagation  FilterDenConstantOutMin=[]  FilterDenConstantOutMax=[]  PCopyOutDataTypeStr=Inherit: Inherit via back propagation  PCopyOutMin=[]  PCopyOutMax=[]  NCopyOutDataTypeStr=Inherit: Inherit via back propagation  NCopyOutMin=[]  NCopyOutMax=[]  IntegratorContinuousStateAttributes=''  IntegratorStateMustResolveToSignalObject=off  IntegratorRTWStateStorageClass=Auto  FilterContinuousStateAttributes=''  FilterStateMustResolveToSignalObject=off  FilterRTWStateStorageClass=Auto  ParallelPVariant=InternalParameters  IdealPVariant=Disabled  IVariant=InternalParameters  DVariant=Disabled  IntegratorVariant=Discrete  SatVariant=Enabled  AWVariant=Passthrough  PCopyVariant=Disabled  TRVariant=Disabled  FdbkBlocksVariant=Forward  IdealPFdbkVariant=Disabled  SatFdbkVariant=Disabled  DerivativeFilterVariant=Disabled  NVariant=Disabled  NCopyVariant=Disabled_SignalSpec  FilterICVariant=Disabled  IntegratorICVariant=InternalICs  ExternalResetVariant=Disabled  TRSumVariant=Passthrough  SumFdbkVariant=Disabled  SumVariant=Sum_PI  TsampFilterVariant=InternalTs  TsampNgainVariant=Passthrough  TsampIntegralVariant=Disabled_SignalSpec  ExternalSaturationOutDataTypeStr=Inherit: Same as second input  DerivativeSourceVariant=Disabled  PreIntVariant=InternalPreInt
  pu->SI2 : Gain  Gain=2/3
  pu->SI3 : Gain  Gain=2/3
  Modulation : PMIOPort  Side=Right
  wires:
  Demux1/2 -> Sum/2  "Qref"
  "Sinusoidal Measurement (PLL, Three-Phase)1"/3 -> Terminator3/1
  Vq Discrete PI Controller/1 -> Mux2/2  "Vq inverter"
  pu->SI3/1 -> Sum/1  "Qmeas"
  Gain/1 -> Discrete-Time Integrator/1
  Reactive power tracking PI contorller/1 -> Sum4/3  "Vd inverter"
  Product2/1 -> Active power tracking PI contorller/1
  Product/1 -> Sum2/2  "Vq_ref"
  Kpf/1 -> Sum5/2
  Demux/2 -> Sum2/1
  Vd Discrete PI Controller/1 -> Mux2/1  "Vd inverter"
  Park Transform/1 -> Demux/1
  Trigonometric Function/1 -> Product/1
  Discrete-Time Integrator/1 -> Trigonometric Function1/1, Trigonometric Function/1
  Product3/1 -> Reactive power tracking PI contorller/1
  FRef/1 -> Sum7/2
  Sum3/1 -> Product2/1, Kpf/1
  Trigonometric Function1/1 -> Product1/2
  Kqv/1 -> Sum4/1
  Sum2/1 -> Vq Discrete PI Controller/1
  Sum1/1 -> Vd Discrete PI Controller/1
  "Sinusoidal Measurement (PLL, Three-Phase)1"/2 -> Inverse Park Transform/2, Park Transform/2
  Mux2/1 -> Inverse Park Transform/1
  Demux/1 -> Sum1/2
  "Sinusoidal Measurement (PLL, Three-Phase)1"/1 -> [freq_mea], Terminator1/1
  "Inverter Active & Reactive Power "/1(P) -> pu->SI2/1  "Inverter Active Power (pu)"
  Product1/1 -> Sum1/1  "Vd_ref"
  [freq_mea] -> Sum7/1
  Sum4/1 -> Product/2, Product1/1
  Demux/3 -> Terminator2/1
  Sum/1 -> Kqv/1, Product3/1
  Bus Element In2/1 -> "Inverter Active & Reactive Power "/2(Iabc)
  Demux1/1 -> Sum3/1  "Pref"
  "Inverter Active & Reactive Power "/2(Q) -> pu->SI3/1  "Inverter Reactive Power (pu)"
  V0/1 -> Mux2/3
  pu->SI2/1 -> Sum3/2
  Bus Element In1/1 -> "Sinusoidal Measurement (PLL, Three-Phase)1"/1
  Bus Element In3/1 -> Park Transform/1
  Bus Element In4/1 -> "Inverter Active & Reactive Power "/1(Vabc)
  Inverse Park Transform/1 -> Unit Delay1/1
  PQref/1 -> Demux1/1
  Unit Delay1/1 -> Simulink-PS Converter2/1
  Sum7/1 -> Sum5/1
  Sum5/1 -> Gain/1
  Active power tracking PI contorller/1 -> Sum7/3
  In Bus Element1/1 -> Active power tracking PI contorller/2
  In Bus Element4/1 -> Reactive power tracking PI contorller/2
  VRef/1 -> Sum4/2
  In Bus Element2/1 -> Product3/2
  In Bus Element3/1 -> Product2/2
  connections:
  Simulink-PS Converter2/RConn1 -- Modulation/RConn1

== system RemoteMicrogrid/Diesel Substation, BESS, & Microgrid Controller/BESS and Controller/BESS Converter Measurement  ==
  Current and Voltage Sensor (Three-Phase) : ee_lib/Sensors & Transducers/Current and Voltage Sensor (Three-Phase)  vMeasurementType=ee.enum.vmeasurement.lg  outputUnit=ee.enum.unit.pu  SRated=150000 A*V  VRated=Microgrid.Voltage V  I_specify=off  I_priority=None  I=[ 0 0 0 ] A  I_nominal_specify=off  I_nominal_value=1  I_nominal_unit=A  V_specify=off  V_priority=None  V=[ 0 0 0 ] V  V_nominal_specify=off  V_nominal_value=1  V_nominal_unit=V
      settings: InternalSimscapePortConfiguration="{\"Bottom\":[],\"Left\":[{\"id\":\"N1\",\"label\":\"~1\",\"type\":\"foundation.electrical.three_phase\"}],\"Right\":[{\"id\":\"V_output\",\"label\":\"V\",\"type\":\"output\"},{\"id\":\"I_output\",\"label\":\"I\",\"type\":\"output\"},{\"id\":\"N2\",\"label\":\"~2\",\"type\":\"foundation.electrical.three_phase\"}],\"Top\":[]}"
  Low-Pass Filter (Discrete or Continuous) : eeGeneralControl/Low-Pass Filter (Discrete or Continuous)  K=1  T=0.02  B=inf  A=-inf  init_option=Inherited from block input  x0=0  Ts=Ts
  Low-Pass Filter (Discrete or Continuous)1 : eeGeneralControl/Low-Pass Filter (Discrete or Continuous)  K=1  T=0.02  B=inf  A=-inf  init_option=Inherited from block input  x0=0  Ts=Ts
  PS-Simulink Converter2 : nesl_utility_internal/PS-Simulink Converter  PhysicalDomain=network_engine_domain  SubClassName=ps_output  LeftPortType=input  RightPortType=output  PseudoPeriodic=off  Frequencies=[]  VectorFormat=1-D array  Unit=V  AffineConversion=off
  PS-Simulink Converter3 : nesl_utility_internal/PS-Simulink Converter  PhysicalDomain=network_engine_domain  SubClassName=ps_output  LeftPortType=input  RightPortType=output  PseudoPeriodic=off  Frequencies=[]  VectorFormat=1-D array  Unit=A  AffineConversion=off
  PS-Simulink Converter6 : nesl_utility_internal/PS-Simulink Converter  PhysicalDomain=network_engine_domain  SubClassName=ps_output  LeftPortType=input  RightPortType=output  PseudoPeriodic=off  Frequencies=[]  VectorFormat=1-D array  Unit=kW  AffineConversion=off
  PS-Simulink Converter7 : nesl_utility_internal/PS-Simulink Converter  PhysicalDomain=network_engine_domain  SubClassName=ps_output  LeftPortType=input  RightPortType=output  PseudoPeriodic=off  Frequencies=[]  VectorFormat=1-D array  Unit=kV*A  AffineConversion=off
  Power Sensor (Three-Phase)1 : ee_lib/Sensors & Transducers/Power Sensor (Three-Phase)  load_type=ee.enum.passive.type_balanced.balanced  f0=60 Hz  config=ee.enum.with_neutral.no  rho=1
      settings: InternalSimscapePortConfiguration="{\"Bottom\":[],\"Left\":[{\"id\":\"N1\",\"label\":\"~1\",\"type\":\"foundation.electrical.three_phase\"}],\"Right\":[{\"id\":\"N2\",\"label\":\"~2\",\"type\":\"foundation.electrical.three_phase\"}],\"Top\":[{\"id\":\"Pm\",\"label\":\"P\",\"type\":\"output\"},{\"id\":\"Qm\",\"label\":\"Q\",\"type\":\"output\"}]}"
  "~ " : PMIOPort  Side=Left
  ~ : PMIOPort  Port=2  Side=Right
  Out Bus Element : Outport  PortName=mBESS  Element=voltage
  Out Bus Element1 : Outport  PortName=mBESS  Element=current
  Out Bus Element2 : Outport  PortName=mBESS  Element=active power
  Out Bus Element3 : Outport  PortName=mBESS  Element=reactive power
  wires:
  PS-Simulink Converter2/1 -> Out Bus Element/1
  PS-Simulink Converter6/1 -> Low-Pass Filter (Discrete or Continuous)1/1
  PS-Simulink Converter7/1 -> Low-Pass Filter (Discrete or Continuous)/1
  PS-Simulink Converter3/1 -> Out Bus Element1/1
  Low-Pass Filter (Discrete or Continuous)/1 -> Out Bus Element3/1
  Low-Pass Filter (Discrete or Continuous)1/1 -> Out Bus Element2/1
  connections:
  Power Sensor (Three-Phase)1/LConn1 -- Current and Voltage Sensor (Three-Phase)/RConn3
  Current and Voltage Sensor (Three-Phase)/LConn1 -- "~ "/RConn1
  PS-Simulink Converter2/LConn1 -- Current and Voltage Sensor (Three-Phase)/RConn1
  Current and Voltage Sensor (Three-Phase)/RConn2 -- PS-Simulink Converter3/LConn1
  Power Sensor (Three-Phase)1/LConn2 -- PS-Simulink Converter6/LConn1
  Power Sensor (Three-Phase)1/LConn3 -- PS-Simulink Converter7/LConn1
  ~/RConn1 -- Power Sensor (Three-Phase)1/RConn1

== system RemoteMicrogrid/Diesel Substation, BESS, & Microgrid Controller/BESS and Controller/BESS Output Filter and Transformer ==
  10 kvar : ee_lib/Passive/RLC Assemblies/Wye-Connected Load  port_option=ee.enum.threePhasePort.composite  parameterization=ee.enum.rlc.parameterization.ratedpower  component_structure=ee.enum.rlc.structure.C  component_structure_PQ=ee.enum.rlc.structure.SeriesRC  R=1 Ohm  L=0.001 H  C=1e-6 F  VRated=Microgrid.Voltage V  FRated=Grid.Frequency Hz  P=1e-4 W  Qpos=0 A*V  Qneg=BESS.Q_BESS_filter A*V  R_parasitic=1e-6 Ohm  G_parasitic=1e-6 1/Ohm  R_parasitic_PQ=1e-6 Ohm  G_parasitic_PQ=1e-6 1/Ohm  Vmag0=0 V  Vang0=0 deg  Freq0=Grid.Frequency Hz  IL_specify=on  IL_priority=High  IL=[ 0 0 0 ] A  IL_nominal_specify=off  IL_nominal_value=1  IL_nominal_unit=A  VC_specify=on  VC_priority=High  VC=[ 0 0 0 ] V  VC_nominal_specify=off  VC_nominal_value=1  VC_nominal_unit=V
  Electrical Reference1 : fl_lib/Electrical/Electrical Elements/Electrical Reference
  Two-Winding Transformer (Three-Phase)1 : ee_lib/Passive/Transformers/Two-Winding Transformer (Three-Phase)  SRated=BESS.TransformerRating A*V  FRated=Grid.Frequency Hz  Winding1Connection=ee.enum.windingconnection.delta11  VRated1=BESS.TransformerPrimaryVoltage V  Winding2Connection=ee.enum.windingconnection.Yg  VRated2=BESS.TransformerSecondaryVoltage V  CoreType=ee.enum.coretype.threelimb  pu_Rw1=BESS.R_BESS_Transformer  pu_Rw2=BESS.R_BESS_Transformer  leakage_reactance_option=ee.enum.transformer_leakage.include  pu_Xl1=BESS.L_BESS_Transformer  pu_Xl2=BESS.L_BESS_Transformer  magnetizing_resistance_option=ee.enum.transformer_magnetizingResistance.include  pu_Rm=500  magnetizing_reactance_option=ee.enum.transformer_magnetizingReactance.include  saturation_option=ee.enum.transformer_saturation.exclude  pu_Xm=500  current_data=[0, .002, 1, 2]  magnetic_flux_data=[0, 1.2, 1.5, 1.51]  pu_X0=0.5  i1_specify=off  i1_priority=None  i1=[0, 0, 0] A  i1_nominal_specify=off  i1_nominal_value=1  i1_nominal_unit=A  i2_specify=off  i2_priority=None  i2=[0, 0, 0] A  i2_nominal_specify=off  i2_nominal_value=1  i2_nominal_unit=A  phi_specify=off  phi_priority=None  phi=[0, 0, 0]  phi_nominal_specify=off  phi_nominal_value=1  phi_nominal_unit=1  power_dissipated_specify=off  power_dissipated_priority=None  power_dissipated=0 W  power_dissipated_nominal_specify=off  power_dissipated_nominal_value=1  power_dissipated_nominal_unit=W
      settings: InternalSimscapePortConfiguration="{\"Bottom\":[],\"Left\":[{\"id\":\"N1\",\"label\":\"~1\",\"type\":\"foundation.electrical.three_phase\"}],\"Right\":[{\"id\":\"N2\",\"label\":\"~2\",\"type\":\"foundation.electrical.three_phase\"}],\"Top\":[]}"
  "~ " : PMIOPort  Side=Right
  ~ : PMIOPort  Port=2  Side=Left
  connections:
  Electrical Reference1/LConn1 -- 10 kvar/RConn1
  ~/RConn1 -- Two-Winding Transformer (Three-Phase)1/LConn1
  Two-Winding Transformer (Three-Phase)1/RConn1 -- "~ "/RConn1 -- 10 kvar/LConn1
